simulink model "model_dyn_ciagly"  (R2023a)
settings: Solver=VariableStepAuto  StartTime=0.0  StopTime=200  RelTol=1e-3
values from neighbouring files (symbols this model uses):
  a0 = 0.000531632    [zad1.m]    (also in zad2_8.m; zadanie_dodatkowe.m)
  a1 = 0.0207337    [zad1.m]    (also in zad2_8.m; zadanie_dodatkowe.m)
  a2 = 0.254652    [zad1.m]    (also in zad2_8.m; zadanie_dodatkowe.m)
  alpha1 = -0.3    [zad1.m]    (also in zad2_8.m; zadanie_dodatkowe.m)
  alpha2 = -0.55    [zad1.m]    (also in zad2_8.m; zadanie_dodatkowe.m)
  alpha3 = 0.4    [zad1.m]    (also in zad2_8.m; zadanie_dodatkowe.m)
  alpha4 = 0.21    [zad1.m]    (also in zad2_8.m; zadanie_dodatkowe.m)
  b0 = 0.00122807    [zad1.m]    (also in zad2_8.m; zadanie_dodatkowe.m)
settings Model: Creator=adams  LastModifiedBy=adams

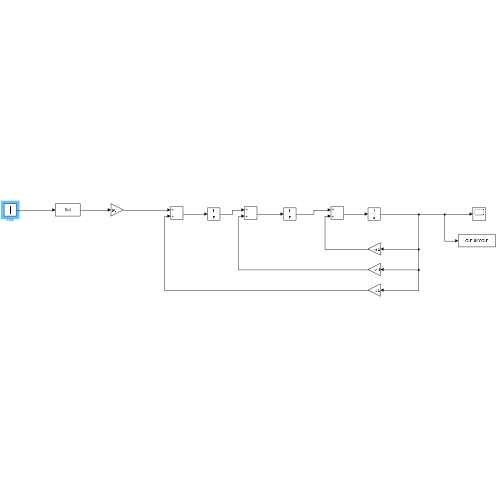
[thumbnail: Simulink's stored preview of the top-level diagram]
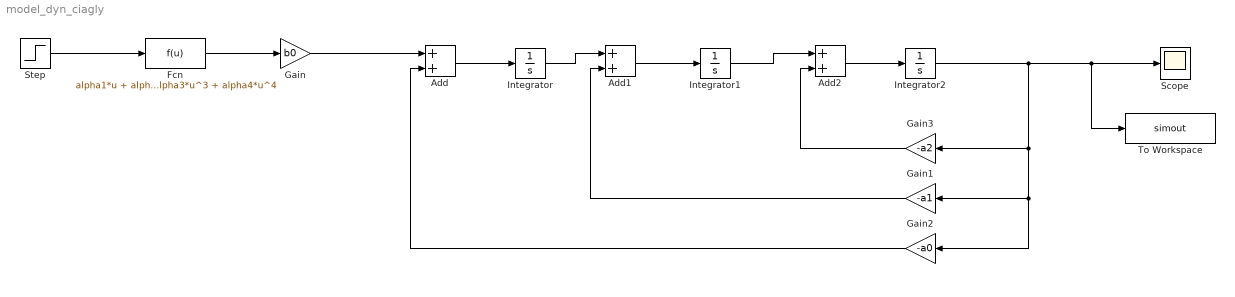
== system model_dyn_ciagly ==
  Add : Sum
  Add1 : Sum
  Add2 : Sum
  Fcn : Fcn  Expr=alpha1*u + alpha2*u^2 + alpha3*u^3 + alpha4*u^4
  Gain : Gain  Gain=b0
  Gain1 : Gain  Gain=-a1
  Gain2 : Gain  Gain=-a0
  Gain3 : Gain  Gain=-a2
  Integrator : Integrator
  Integrator1 : Integrator
  Integrator2 : Integrator
  Scope : Scope
  Step : Step  SampleTime=0
  To Workspace : ToWorkspace  VariableName=simout  SaveFormat=Structure With Time  SampleTime=-1
  wires:
  Integrator2/1 -> Gain1/1, Gain2/1, Gain3/1, To Workspace/1, Scope/1
  Fcn/1 -> Gain/1
  Add/1 -> Integrator/1
  Gain/1 -> Add/1
  Gain2/1 -> Add/2
  Integrator/1 -> Add1/1
  Add1/1 -> Integrator1/1
  Gain1/1 -> Add1/2
  Integrator1/1 -> Add2/1
  Gain3/1 -> Add2/2
  Add2/1 -> Integrator2/1
  Step/1 -> Fcn/1
